simulink model "FaultModel (1)"  (R2018b)
settings: Solver=VariableStepAuto  StartTime=0.0  StopTime=0.05  RelTol=1e-3
undefined symbols (not defined in the file or in its folder): D1, Delta
libraries: powerlib x316
(part 2 of 4)

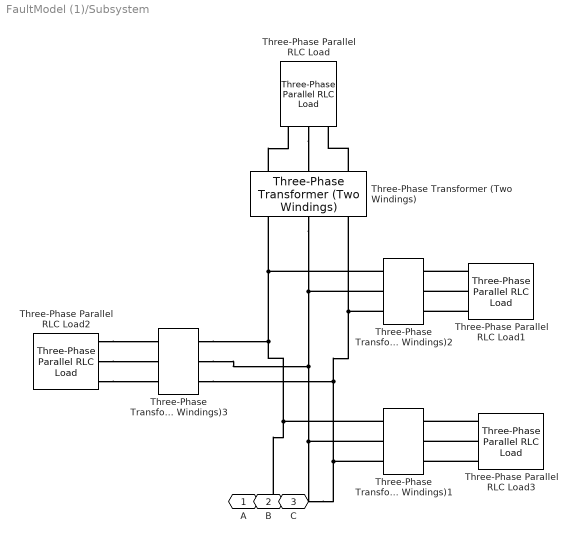
== system FaultModel (1)/Subsystem ==
  Three-Phase Parallel RLC Load{,1..3} (4 alike) : powerlib/Elements/Three-Phase Parallel RLC Load  LConnTagsString=A|B|C  Configuration=Y (grounded)  NominalVoltage=33e3  Vabc=[1e3 1e3 1e3]  Vabcp=[1e3 1e3 1e3]  NominalFrequency=50  UnbalancedPower=off  ActivePower=32.8e6  InductivePower=100  CapacitivePower=100  Pabc=[10e3 9e3 11e3]  QLabc=[100 90 110]  QCabc=[100 90 110]  Pabcp=[10e3 9e3 11e3]  QLabcp=[100 90 110]  QCabcp=[100 90 110]  Measurements=None  LoadType=constant Z
  Three-Phase Transformer (Two Windings){,1..3} (4 alike) : powerlib/Elements/Three-Phase Transformer (Two Windings)  Winding1Connection=Delta (D1)  Winding2Connection=Yg  CoreType=Three single-phase transformers  SetSaturation=off  Hysteresis=off  DataFile='hysteresis'  SetInitialFlux=off  Measurements=None  UNITS=pu  NominalPower=[ 41e6 , 50 ]  Winding1=[ 132e3 , 0.002 , 0.08 ]  Winding2=[ 33e3 , 0.002 , 0.08 ]  Rm=500  Lm=500  L0=0.5  Saturation=[ 0,0 ; 0.0024,1.2 ; 1.0,1.52 ]  InitialFluxes=[ 0.8 , -0.8 , 0.7 ]  BreakLoop=off  DiscreteSolver=Trapezoidal iterative  DataType=off  TransfoNumber=1
  A : PMIOPort  Side=Left
  B : PMIOPort  Port=2  Side=Left
  C : PMIOPort  Port=3  Side=Left
  connections:
  Three-Phase Parallel RLC Load2/LConn3 -- Three-Phase Transformer (Two Windings)3/RConn3
  Three-Phase Parallel RLC Load1/LConn1 -- Three-Phase Transformer (Two Windings)2/RConn1
  Three-Phase Parallel RLC Load1/LConn2 -- Three-Phase Transformer (Two Windings)2/RConn2
  Three-Phase Transformer (Two Windings)1/LConn3 -- C/RConn1 -- Three-Phase Transformer (Two Windings)3/LConn3 -- Three-Phase Transformer (Two Windings)2/LConn3 -- Three-Phase Transformer (Two Windings)/LConn3
  Three-Phase Transformer (Two Windings)/LConn2 -- Three-Phase Transformer (Two Windings)2/LConn2 -- Three-Phase Transformer (Two Windings)3/LConn2 -- B/RConn1 -- Three-Phase Transformer (Two Windings)1/LConn2
  Three-Phase Parallel RLC Load3/LConn2 -- Three-Phase Transformer (Two Windings)1/RConn2
  Three-Phase Transformer (Two Windings)1/LConn1 -- A/RConn1 -- Three-Phase Transformer (Two Windings)3/LConn1 -- Three-Phase Transformer (Two Windings)2/LConn1 -- Three-Phase Transformer (Two Windings)/LConn1
  Three-Phase Parallel RLC Load/LConn2 -- Three-Phase Transformer (Two Windings)/RConn2
  Three-Phase Parallel RLC Load2/LConn2 -- Three-Phase Transformer (Two Windings)3/RConn2
  Three-Phase Transformer (Two Windings)/RConn1 -- Three-Phase Parallel RLC Load/LConn1
  Three-Phase Transformer (Two Windings)/RConn3 -- Three-Phase Parallel RLC Load/LConn3
  Three-Phase Parallel RLC Load2/LConn1 -- Three-Phase Transformer (Two Windings)3/RConn1
  Three-Phase Parallel RLC Load3/LConn3 -- Three-Phase Transformer (Two Windings)1/RConn3
  Three-Phase Parallel RLC Load3/LConn1 -- Three-Phase Transformer (Two Windings)1/RConn1
  Three-Phase Parallel RLC Load1/LConn3 -- Three-Phase Transformer (Two Windings)2/RConn3

== system FaultModel (1)/Subsystem1 ==
  Three-Phase Parallel RLC Load4 : powerlib/Elements/Three-Phase Parallel RLC Load  LConnTagsString=A|B|C  Configuration=Y (grounded)  NominalVoltage=33e3  Vabc=[1e3 1e3 1e3]  Vabcp=[1e3 1e3 1e3]  NominalFrequency=50  UnbalancedPower=off  ActivePower=60e6  InductivePower=100  CapacitivePower=100  Pabc=[10e3 9e3 11e3]  QLabc=[100 90 110]  QCabc=[100 90 110]  Pabcp=[10e3 9e3 11e3]  QLabcp=[100 90 110]  QCabcp=[100 90 110]  Measurements=None  LoadType=constant Z
  Three-Phase Parallel RLC Load5 : powerlib/Elements/Three-Phase Parallel RLC Load  LConnTagsString=A|B|C  Configuration=Y (grounded)  NominalVoltage=33e3  Vabc=[1e3 1e3 1e3]  Vabcp=[1e3 1e3 1e3]  NominalFrequency=50  UnbalancedPower=off  ActivePower=60e6  InductivePower=100  CapacitivePower=100  Pabc=[10e3 9e3 11e3]  QLabc=[100 90 110]  QCabc=[100 90 110]  Pabcp=[10e3 9e3 11e3]  QLabcp=[100 90 110]  QCabcp=[100 90 110]  Measurements=None  LoadType=constant Z
  Three-Phase Transformer (Two Windings)4 : powerlib/Elements/Three-Phase Transformer (Two Windings)  Winding1Connection=Delta (D1)  Winding2Connection=Yg  CoreType=Three single-phase transformers  SetSaturation=off  Hysteresis=off  DataFile='hysteresis'  SetInitialFlux=off  Measurements=None  UNITS=pu  NominalPower=[ 75e6 , 50 ]  Winding1=[ 132e3 , 0.002 , 0.08 ]  Winding2=[ 33e3 , 0.002 , 0.08 ]  Rm=500  Lm=500  L0=0.5  Saturation=[ 0,0 ; 0.0024,1.2 ; 1.0,1.52 ]  InitialFluxes=[ 0.8 , -0.8 , 0.7 ]  BreakLoop=off  DiscreteSolver=Trapezoidal iterative  DataType=off  TransfoNumber=1
  Three-Phase Transformer (Two Windings)5 : powerlib/Elements/Three-Phase Transformer (Two Windings)  Winding1Connection=Delta (D1)  Winding2Connection=Yg  CoreType=Three single-phase transformers  SetSaturation=off  Hysteresis=off  DataFile='hysteresis'  SetInitialFlux=off  Measurements=None  UNITS=pu  NominalPower=[ 75e6 , 50 ]  Winding1=[ 132e3 , 0.002 , 0.08 ]  Winding2=[ 33e3 , 0.002 , 0.08 ]  Rm=500  Lm=500  L0=0.5  Saturation=[ 0,0 ; 0.0024,1.2 ; 1.0,1.52 ]  InitialFluxes=[ 0.8 , -0.8 , 0.7 ]  BreakLoop=off  DiscreteSolver=Trapezoidal iterative  DataType=off  TransfoNumber=1
  A : PMIOPort  Side=Left
  B : PMIOPort  Port=2  Side=Left
  C : PMIOPort  Port=3  Side=Left
  connections:
  Three-Phase Parallel RLC Load4/LConn2 -- Three-Phase Transformer (Two Windings)5/RConn2
  Three-Phase Parallel RLC Load5/LConn1 -- Three-Phase Transformer (Two Windings)4/RConn1
  Three-Phase Transformer (Two Windings)5/LConn3 -- C/RConn1 -- Three-Phase Transformer (Two Windings)4/LConn3
  Three-Phase Transformer (Two Windings)4/LConn2 -- B/RConn1 -- Three-Phase Transformer (Two Windings)5/LConn2
  Three-Phase Parallel RLC Load4/LConn1 -- Three-Phase Transformer (Two Windings)5/RConn1
  Three-Phase Transformer (Two Windings)4/LConn1 -- A/RConn1 -- Three-Phase Transformer (Two Windings)5/LConn1
  Three-Phase Parallel RLC Load5/LConn2 -- Three-Phase Transformer (Two Windings)4/RConn2
  Three-Phase Parallel RLC Load5/LConn3 -- Three-Phase Transformer (Two Windings)4/RConn3
  Three-Phase Parallel RLC Load4/LConn3 -- Three-Phase Transformer (Two Windings)5/RConn3

== system FaultModel (1)/Subsystem10 ==
  Three-Phase Parallel RLC Load34 : powerlib/Elements/Three-Phase Parallel RLC Load  LConnTagsString=A|B|C  Configuration=Y (grounded)  NominalVoltage=33e3  Vabc=[1e3 1e3 1e3]  Vabcp=[1e3 1e3 1e3]  NominalFrequency=50  UnbalancedPower=off  ActivePower=96e6  InductivePower=100  CapacitivePower=100  Pabc=[10e3 9e3 11e3]  QLabc=[100 90 110]  QCabc=[100 90 110]  Pabcp=[10e3 9e3 11e3]  QLabcp=[100 90 110]  QCabcp=[100 90 110]  Measurements=None  LoadType=constant Z
  Three-Phase Parallel RLC Load35 : powerlib/Elements/Three-Phase Parallel RLC Load  LConnTagsString=A|B|C  Configuration=Y (grounded)  NominalVoltage=33e3  Vabc=[1e3 1e3 1e3]  Vabcp=[1e3 1e3 1e3]  NominalFrequency=50  UnbalancedPower=off  ActivePower=96e6  InductivePower=100  CapacitivePower=100  Pabc=[10e3 9e3 11e3]  QLabc=[100 90 110]  QCabc=[100 90 110]  Pabcp=[10e3 9e3 11e3]  QLabcp=[100 90 110]  QCabcp=[100 90 110]  Measurements=None  LoadType=constant Z
  Three-Phase Transformer (Two Windings)34 : powerlib/Elements/Three-Phase Transformer (Two Windings)  Winding1Connection=Delta (D1)  Winding2Connection=Yg  CoreType=Three single-phase transformers  SetSaturation=off  Hysteresis=off  DataFile='hysteresis'  SetInitialFlux=off  Measurements=None  UNITS=pu  NominalPower=[120e6 , 50 ]  Winding1=[ 132e3 , 0.002 , 0.08 ]  Winding2=[ 33e3 , 0.002 , 0.08 ]  Rm=500  Lm=500  L0=0.5  Saturation=[ 0,0 ; 0.0024,1.2 ; 1.0,1.52 ]  InitialFluxes=[ 0.8 , -0.8 , 0.7 ]  BreakLoop=off  DiscreteSolver=Trapezoidal iterative  DataType=off  TransfoNumber=1
  Three-Phase Transformer (Two Windings)35 : powerlib/Elements/Three-Phase Transformer (Two Windings)  Winding1Connection=Delta (D1)  Winding2Connection=Yg  CoreType=Three single-phase transformers  SetSaturation=off  Hysteresis=off  DataFile='hysteresis'  SetInitialFlux=off  Measurements=None  UNITS=pu  NominalPower=[120e6 , 50 ]  Winding1=[ 132e3 , 0.002 , 0.08 ]  Winding2=[ 33e3 , 0.002 , 0.08 ]  Rm=500  Lm=500  L0=0.5  Saturation=[ 0,0 ; 0.0024,1.2 ; 1.0,1.52 ]  InitialFluxes=[ 0.8 , -0.8 , 0.7 ]  BreakLoop=off  DiscreteSolver=Trapezoidal iterative  DataType=off  TransfoNumber=1
  A : PMIOPort  Side=Left
  B : PMIOPort  Port=2  Side=Left
  C : PMIOPort  Port=3  Side=Left
  connections:
  Three-Phase Parallel RLC Load35/LConn3 -- Three-Phase Transformer (Two Windings)35/RConn3
  Three-Phase Transformer (Two Windings)34/LConn3 -- C/RConn1 -- Three-Phase Transformer (Two Windings)35/LConn3
  Three-Phase Parallel RLC Load34/LConn2 -- Three-Phase Transformer (Two Windings)34/RConn2
  Three-Phase Transformer (Two Windings)34/LConn2 -- B/RConn1 -- Three-Phase Transformer (Two Windings)35/LConn2
  Three-Phase Parallel RLC Load34/LConn3 -- Three-Phase Transformer (Two Windings)34/RConn3
  Three-Phase Parallel RLC Load35/LConn2 -- Three-Phase Transformer (Two Windings)35/RConn2
  Three-Phase Parallel RLC Load35/LConn1 -- Three-Phase Transformer (Two Windings)35/RConn1
  Three-Phase Parallel RLC Load34/LConn1 -- Three-Phase Transformer (Two Windings)34/RConn1
  Three-Phase Transformer (Two Windings)34/LConn1 -- A/RConn1 -- Three-Phase Transformer (Two Windings)35/LConn1

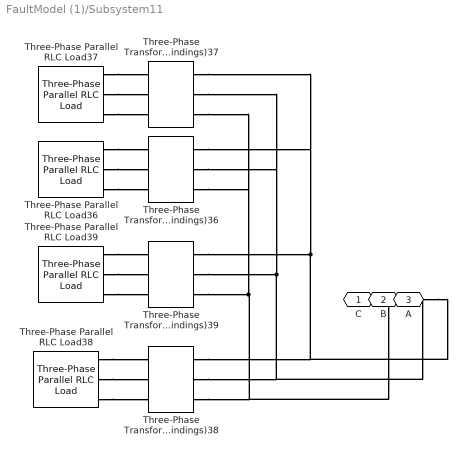
== system FaultModel (1)/Subsystem11 ==
  Three-Phase Parallel RLC Load{36..39} (4 alike) : powerlib/Elements/Three-Phase Parallel RLC Load  LConnTagsString=A|B|C  Configuration=Y (grounded)  NominalVoltage=33e3  Vabc=[1e3 1e3 1e3]  Vabcp=[1e3 1e3 1e3]  NominalFrequency=50  UnbalancedPower=off  ActivePower=32.8e6  InductivePower=100  CapacitivePower=100  Pabc=[10e3 9e3 11e3]  QLabc=[100 90 110]  QCabc=[100 90 110]  Pabcp=[10e3 9e3 11e3]  QLabcp=[100 90 110]  QCabcp=[100 90 110]  Measurements=None  LoadType=constant Z
  Three-Phase Transformer (Two Windings){36..39} (4 alike) : powerlib/Elements/Three-Phase Transformer (Two Windings)  Winding1Connection=Delta (D1)  Winding2Connection=Yg  CoreType=Three single-phase transformers  SetSaturation=off  Hysteresis=off  DataFile='hysteresis'  SetInitialFlux=off  Measurements=None  UNITS=pu  NominalPower=[41e6 , 50 ]  Winding1=[ 132e3 , 0.002 , 0.08 ]  Winding2=[ 33e3 , 0.002 , 0.08 ]  Rm=500  Lm=500  L0=0.5  Saturation=[ 0,0 ; 0.0024,1.2 ; 1.0,1.52 ]  InitialFluxes=[ 0.8 , -0.8 , 0.7 ]  BreakLoop=off  DiscreteSolver=Trapezoidal iterative  DataType=off  TransfoNumber=1
  C : PMIOPort  Side=Left
  B : PMIOPort  Port=2  Side=Left
  A : PMIOPort  Port=3  Side=Left
  connections:
  Three-Phase Transformer (Two Windings)39/LConn1 -- Three-Phase Transformer (Two Windings)37/LConn1 -- Three-Phase Transformer (Two Windings)36/LConn1 -- A/RConn1 -- Three-Phase Transformer (Two Windings)38/LConn1
  Three-Phase Parallel RLC Load38/LConn3 -- Three-Phase Transformer (Two Windings)38/RConn3
  Three-Phase Parallel RLC Load36/LConn3 -- Three-Phase Transformer (Two Windings)36/RConn3
  Three-Phase Parallel RLC Load36/LConn1 -- Three-Phase Transformer (Two Windings)36/RConn1
  Three-Phase Parallel RLC Load37/LConn1 -- Three-Phase Transformer (Two Windings)37/RConn1
  Three-Phase Transformer (Two Windings)39/LConn3 -- Three-Phase Transformer (Two Windings)37/LConn3 -- Three-Phase Transformer (Two Windings)36/LConn3 -- C/RConn1 -- Three-Phase Transformer (Two Windings)38/LConn3
  Three-Phase Parallel RLC Load37/LConn3 -- Three-Phase Transformer (Two Windings)37/RConn3
  Three-Phase Transformer (Two Windings)39/LConn2 -- Three-Phase Transformer (Two Windings)37/LConn2 -- Three-Phase Transformer (Two Windings)36/LConn2 -- B/RConn1 -- Three-Phase Transformer (Two Windings)38/LConn2
  Three-Phase Parallel RLC Load39/LConn1 -- Three-Phase Transformer (Two Windings)39/RConn1
  Three-Phase Parallel RLC Load38/LConn2 -- Three-Phase Transformer (Two Windings)38/RConn2
  Three-Phase Parallel RLC Load38/LConn1 -- Three-Phase Transformer (Two Windings)38/RConn1
  Three-Phase Parallel RLC Load39/LConn2 -- Three-Phase Transformer (Two Windings)39/RConn2
  Three-Phase Parallel RLC Load36/LConn2 -- Three-Phase Transformer (Two Windings)36/RConn2
  Three-Phase Parallel RLC Load37/LConn2 -- Three-Phase Transformer (Two Windings)37/RConn2
  Three-Phase Parallel RLC Load39/LConn3 -- Three-Phase Transformer (Two Windings)39/RConn3

== system FaultModel (1)/Subsystem12 ==
  Three-Phase Parallel RLC Load40 : powerlib/Elements/Three-Phase Parallel RLC Load  LConnTagsString=A|B|C  Configuration=Y (grounded)  NominalVoltage=33e3  Vabc=[1e3 1e3 1e3]  Vabcp=[1e3 1e3 1e3]  NominalFrequency=50  UnbalancedPower=off  ActivePower=32.8e6  InductivePower=100  CapacitivePower=100  Pabc=[10e3 9e3 11e3]  QLabc=[100 90 110]  QCabc=[100 90 110]  Pabcp=[10e3 9e3 11e3]  QLabcp=[100 90 110]  QCabcp=[100 90 110]  Measurements=None  LoadType=constant Z
  Three-Phase Parallel RLC Load41 : powerlib/Elements/Three-Phase Parallel RLC Load  LConnTagsString=A|B|C  Configuration=Y (grounded)  NominalVoltage=33e3  Vabc=[1e3 1e3 1e3]  Vabcp=[1e3 1e3 1e3]  NominalFrequency=50  UnbalancedPower=off  ActivePower=40e6  InductivePower=100  CapacitivePower=100  Pabc=[10e3 9e3 11e3]  QLabc=[100 90 110]  QCabc=[100 90 110]  Pabcp=[10e3 9e3 11e3]  QLabcp=[100 90 110]  QCabcp=[100 90 110]  Measurements=None  LoadType=constant Z
  Three-Phase Parallel RLC Load42 : powerlib/Elements/Three-Phase Parallel RLC Load  LConnTagsString=A|B|C  Configuration=Y (grounded)  NominalVoltage=33e3  Vabc=[1e3 1e3 1e3]  Vabcp=[1e3 1e3 1e3]  NominalFrequency=50  UnbalancedPower=off  ActivePower=40e6  InductivePower=100  CapacitivePower=100  Pabc=[10e3 9e3 11e3]  QLabc=[100 90 110]  QCabc=[100 90 110]  Pabcp=[10e3 9e3 11e3]  QLabcp=[100 90 110]  QCabcp=[100 90 110]  Measurements=None  LoadType=constant Z
  Three-Phase Transformer (Two Windings)40 : powerlib/Elements/Three-Phase Transformer (Two Windings)  Winding1Connection=Delta (D1)  Winding2Connection=Yg  CoreType=Three single-phase transformers  SetSaturation=off  Hysteresis=off  DataFile='hysteresis'  SetInitialFlux=off  Measurements=None  UNITS=pu  NominalPower=[41e6 , 50 ]  Winding1=[ 132e3 , 0.002 , 0.08 ]  Winding2=[ 33e3 , 0.002 , 0.08 ]  Rm=500  Lm=500  L0=0.5  Saturation=[ 0,0 ; 0.0024,1.2 ; 1.0,1.52 ]  InitialFluxes=[ 0.8 , -0.8 , 0.7 ]  BreakLoop=off  DiscreteSolver=Trapezoidal iterative  DataType=off  TransfoNumber=1
  Three-Phase Transformer (Two Windings)41 : powerlib/Elements/Three-Phase Transformer (Two Windings)  Winding1Connection=Delta (D1)  Winding2Connection=Yg  CoreType=Three single-phase transformers  SetSaturation=off  Hysteresis=off  DataFile='hysteresis'  SetInitialFlux=off  Measurements=None  UNITS=pu  NominalPower=[50e6 , 50 ]  Winding1=[ 132e3 , 0.002 , 0.08 ]  Winding2=[ 33e3 , 0.002 , 0.08 ]  Rm=500  Lm=500  L0=0.5  Saturation=[ 0,0 ; 0.0024,1.2 ; 1.0,1.52 ]  InitialFluxes=[ 0.8 , -0.8 , 0.7 ]  BreakLoop=off  DiscreteSolver=Trapezoidal iterative  DataType=off  TransfoNumber=1
  Three-Phase Transformer (Two Windings)42 : powerlib/Elements/Three-Phase Transformer (Two Windings)  Winding1Connection=Delta (D1)  Winding2Connection=Yg  CoreType=Three single-phase transformers  SetSaturation=off  Hysteresis=off  DataFile='hysteresis'  SetInitialFlux=off  Measurements=None  UNITS=pu  NominalPower=[50e6 , 50 ]  Winding1=[ 132e3 , 0.002 , 0.08 ]  Winding2=[ 33e3 , 0.002 , 0.08 ]  Rm=500  Lm=500  L0=0.5  Saturation=[ 0,0 ; 0.0024,1.2 ; 1.0,1.52 ]  InitialFluxes=[ 0.8 , -0.8 , 0.7 ]  BreakLoop=off  DiscreteSolver=Trapezoidal iterative  DataType=off  TransfoNumber=1
  A : PMIOPort  Side=Left
  B : PMIOPort  Port=2  Side=Left
  C : PMIOPort  Port=3  Side=Left
  connections:
  Three-Phase Parallel RLC Load40/LConn2 -- Three-Phase Transformer (Two Windings)40/RConn2
  Three-Phase Parallel RLC Load42/LConn2 -- Three-Phase Transformer (Two Windings)42/RConn2
  Three-Phase Transformer (Two Windings)42/LConn2 -- Three-Phase Transformer (Two Windings)41/LConn2 -- Three-Phase Transformer (Two Windings)40/LConn2 -- B/RConn1
  Three-Phase Transformer (Two Windings)41/LConn3 -- Three-Phase Transformer (Two Windings)42/LConn3 -- C/RConn1 -- Three-Phase Transformer (Two Windings)40/LConn3
  Three-Phase Parallel RLC Load40/LConn1 -- Three-Phase Transformer (Two Windings)40/RConn1
  Three-Phase Parallel RLC Load41/LConn2 -- Three-Phase Transformer (Two Windings)41/RConn2
  Three-Phase Parallel RLC Load40/LConn3 -- Three-Phase Transformer (Two Windings)40/RConn3
  Three-Phase Parallel RLC Load42/LConn1 -- Three-Phase Transformer (Two Windings)42/RConn1
  Three-Phase Parallel RLC Load41/LConn3 -- Three-Phase Transformer (Two Windings)41/RConn3
  Three-Phase Parallel RLC Load42/LConn3 -- Three-Phase Transformer (Two Windings)42/RConn3
  Three-Phase Transformer (Two Windings)42/LConn1 -- A/RConn1 -- Three-Phase Transformer (Two Windings)41/LConn1 -- Three-Phase Transformer (Two Windings)40/LConn1
  Three-Phase Parallel RLC Load41/LConn1 -- Three-Phase Transformer (Two Windings)41/RConn1

== system FaultModel (1)/Subsystem13 ==
  Three-Phase Parallel RLC Load43 : powerlib/Elements/Three-Phase Parallel RLC Load  LConnTagsString=A|B|C  Configuration=Y (grounded)  NominalVoltage=33e3  Vabc=[1e3 1e3 1e3]  Vabcp=[1e3 1e3 1e3]  NominalFrequency=50  UnbalancedPower=off  ActivePower=60e6  InductivePower=100  CapacitivePower=100  Pabc=[10e3 9e3 11e3]  QLabc=[100 90 110]  QCabc=[100 90 110]  Pabcp=[10e3 9e3 11e3]  QLabcp=[100 90 110]  QCabcp=[100 90 110]  Measurements=None  LoadType=constant Z
  Three-Phase Parallel RLC Load44 : powerlib/Elements/Three-Phase Parallel RLC Load  LConnTagsString=A|B|C  Configuration=Y (grounded)  NominalVoltage=33e3  Vabc=[1e3 1e3 1e3]  Vabcp=[1e3 1e3 1e3]  NominalFrequency=50  UnbalancedPower=off  ActivePower=60e6  InductivePower=100  CapacitivePower=100  Pabc=[10e3 9e3 11e3]  QLabc=[100 90 110]  QCabc=[100 90 110]  Pabcp=[10e3 9e3 11e3]  QLabcp=[100 90 110]  QCabcp=[100 90 110]  Measurements=None  LoadType=constant Z
  Three-Phase Parallel RLC Load45 : powerlib/Elements/Three-Phase Parallel RLC Load  LConnTagsString=A|B|C  Configuration=Y (grounded)  NominalVoltage=33e3  Vabc=[1e3 1e3 1e3]  Vabcp=[1e3 1e3 1e3]  NominalFrequency=50  UnbalancedPower=off  ActivePower=60e6  InductivePower=100  CapacitivePower=100  Pabc=[10e3 9e3 11e3]  QLabc=[100 90 110]  QCabc=[100 90 110]  Pabcp=[10e3 9e3 11e3]  QLabcp=[100 90 110]  QCabcp=[100 90 110]  Measurements=None  LoadType=constant Z
  Three-Phase Transformer (Two Windings)43 : powerlib/Elements/Three-Phase Transformer (Two Windings)  Winding1Connection=Delta (D1)  Winding2Connection=Yg  CoreType=Three single-phase transformers  SetSaturation=off  Hysteresis=off  DataFile='hysteresis'  SetInitialFlux=off  Measurements=None  UNITS=pu  NominalPower=[75e6 , 50 ]  Winding1=[ 132e3 , 0.002 , 0.08 ]  Winding2=[ 33e3 , 0.002 , 0.08 ]  Rm=500  Lm=500  L0=0.5  Saturation=[ 0,0 ; 0.0024,1.2 ; 1.0,1.52 ]  InitialFluxes=[ 0.8 , -0.8 , 0.7 ]  BreakLoop=off  DiscreteSolver=Trapezoidal iterative  DataType=off  TransfoNumber=1
  Three-Phase Transformer (Two Windings)44 : powerlib/Elements/Three-Phase Transformer (Two Windings)  Winding1Connection=Delta (D1)  Winding2Connection=Yg  CoreType=Three single-phase transformers  SetSaturation=off  Hysteresis=off  DataFile='hysteresis'  SetInitialFlux=off  Measurements=None  UNITS=pu  NominalPower=[75e6 , 50 ]  Winding1=[ 132e3 , 0.002 , 0.08 ]  Winding2=[ 33e3 , 0.002 , 0.08 ]  Rm=500  Lm=500  L0=0.5  Saturation=[ 0,0 ; 0.0024,1.2 ; 1.0,1.52 ]  InitialFluxes=[ 0.8 , -0.8 , 0.7 ]  BreakLoop=off  DiscreteSolver=Trapezoidal iterative  DataType=off  TransfoNumber=1
  Three-Phase Transformer (Two Windings)45 : powerlib/Elements/Three-Phase Transformer (Two Windings)  Winding1Connection=Delta (D1)  Winding2Connection=Yg  CoreType=Three single-phase transformers  SetSaturation=off  Hysteresis=off  DataFile='hysteresis'  SetInitialFlux=off  Measurements=None  UNITS=pu  NominalPower=[75e6 , 50 ]  Winding1=[ 132e3 , 0.002 , 0.08 ]  Winding2=[ 33e3 , 0.002 , 0.08 ]  Rm=500  Lm=500  L0=0.5  Saturation=[ 0,0 ; 0.0024,1.2 ; 1.0,1.52 ]  InitialFluxes=[ 0.8 , -0.8 , 0.7 ]  BreakLoop=off  DiscreteSolver=Trapezoidal iterative  DataType=off  TransfoNumber=1
  A : PMIOPort  Side=Left
  B : PMIOPort  Port=2  Side=Left
  C : PMIOPort  Port=3  Side=Left
  connections:
  Three-Phase Parallel RLC Load43/LConn3 -- Three-Phase Transformer (Two Windings)43/RConn3
  Three-Phase Transformer (Two Windings)43/LConn2 -- B/RConn1 -- Three-Phase Transformer (Two Windings)44/LConn2 -- Three-Phase Transformer (Two Windings)45/LConn2
  Three-Phase Parallel RLC Load43/LConn2 -- Three-Phase Transformer (Two Windings)43/RConn2
  Three-Phase Transformer (Two Windings)43/LConn1 -- A/RConn1 -- Three-Phase Transformer (Two Windings)44/LConn1 -- Three-Phase Transformer (Two Windings)45/LConn1
  Three-Phase Transformer (Two Windings)43/LConn3 -- C/RConn1 -- Three-Phase Transformer (Two Windings)44/LConn3 -- Three-Phase Transformer (Two Windings)45/LConn3
  Three-Phase Parallel RLC Load44/LConn1 -- Three-Phase Transformer (Two Windings)44/RConn1
  Three-Phase Parallel RLC Load43/LConn1 -- Three-Phase Transformer (Two Windings)43/RConn1
  Three-Phase Parallel RLC Load45/LConn1 -- Three-Phase Transformer (Two Windings)45/RConn1
  Three-Phase Parallel RLC Load44/LConn2 -- Three-Phase Transformer (Two Windings)44/RConn2
  Three-Phase Parallel RLC Load45/LConn3 -- Three-Phase Transformer (Two Windings)45/RConn3
  Three-Phase Parallel RLC Load44/LConn3 -- Three-Phase Transformer (Two Windings)44/RConn3
  Three-Phase Parallel RLC Load45/LConn2 -- Three-Phase Transformer (Two Windings)45/RConn2

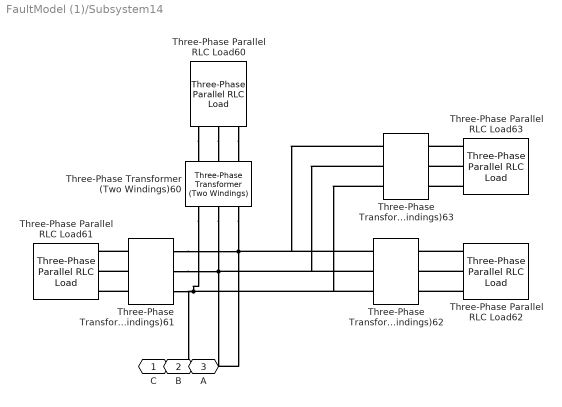
== system FaultModel (1)/Subsystem14 ==
  Three-Phase Parallel RLC Load60 : powerlib/Elements/Three-Phase Parallel RLC Load  LConnTagsString=A|B|C  Configuration=Y (grounded)  NominalVoltage=33e3  Vabc=[1e3 1e3 1e3]  Vabcp=[1e3 1e3 1e3]  NominalFrequency=50  UnbalancedPower=off  ActivePower=60e6  InductivePower=100  CapacitivePower=100  Pabc=[10e3 9e3 11e3]  QLabc=[100 90 110]  QCabc=[100 90 110]  Pabcp=[10e3 9e3 11e3]  QLabcp=[100 90 110]  QCabcp=[100 90 110]  Measurements=None  LoadType=constant Z
  Three-Phase Parallel RLC Load61 : powerlib/Elements/Three-Phase Parallel RLC Load  LConnTagsString=A|B|C  Configuration=Y (grounded)  NominalVoltage=33e3  Vabc=[1e3 1e3 1e3]  Vabcp=[1e3 1e3 1e3]  NominalFrequency=50  UnbalancedPower=off  ActivePower=60e6  InductivePower=100  CapacitivePower=100  Pabc=[10e3 9e3 11e3]  QLabc=[100 90 110]  QCabc=[100 90 110]  Pabcp=[10e3 9e3 11e3]  QLabcp=[100 90 110]  QCabcp=[100 90 110]  Measurements=None  LoadType=constant Z
  Three-Phase Parallel RLC Load62 : powerlib/Elements/Three-Phase Parallel RLC Load  LConnTagsString=A|B|C  Configuration=Y (grounded)  NominalVoltage=33e3  Vabc=[1e3 1e3 1e3]  Vabcp=[1e3 1e3 1e3]  NominalFrequency=50  UnbalancedPower=off  ActivePower=32.8e6  InductivePower=100  CapacitivePower=100  Pabc=[10e3 9e3 11e3]  QLabc=[100 90 110]  QCabc=[100 90 110]  Pabcp=[10e3 9e3 11e3]  QLabcp=[100 90 110]  QCabcp=[100 90 110]  Measurements=None  LoadType=constant Z
  Three-Phase Parallel RLC Load63 : powerlib/Elements/Three-Phase Parallel RLC Load  LConnTagsString=A|B|C  Configuration=Y (grounded)  NominalVoltage=33e3  Vabc=[1e3 1e3 1e3]  Vabcp=[1e3 1e3 1e3]  NominalFrequency=50  UnbalancedPower=off  ActivePower=16e6  InductivePower=100  CapacitivePower=100  Pabc=[10e3 9e3 11e3]  QLabc=[100 90 110]  QCabc=[100 90 110]  Pabcp=[10e3 9e3 11e3]  QLabcp=[100 90 110]  QCabcp=[100 90 110]  Measurements=None  LoadType=constant Z
  Three-Phase Transformer (Two Windings)60 : powerlib/Elements/Three-Phase Transformer (Two Windings)  Winding1Connection=Delta (D1)  Winding2Connection=Yg  CoreType=Three single-phase transformers  SetSaturation=off  Hysteresis=off  DataFile='hysteresis'  SetInitialFlux=off  Measurements=None  UNITS=pu  NominalPower=[75e6 , 50 ]  Winding1=[ 132e3 , 0.002 , 0.08 ]  Winding2=[ 33e3 , 0.002 , 0.08 ]  Rm=500  Lm=500  L0=0.5  Saturation=[ 0,0 ; 0.0024,1.2 ; 1.0,1.52 ]  InitialFluxes=[ 0.8 , -0.8 , 0.7 ]  BreakLoop=off  DiscreteSolver=Trapezoidal iterative  DataType=off  TransfoNumber=1
  Three-Phase Transformer (Two Windings)61 : powerlib/Elements/Three-Phase Transformer (Two Windings)  Winding1Connection=Delta (D1)  Winding2Connection=Yg  CoreType=Three single-phase transformers  SetSaturation=off  Hysteresis=off  DataFile='hysteresis'  SetInitialFlux=off  Measurements=None  UNITS=pu  NominalPower=[75e6 , 50 ]  Winding1=[ 132e3 , 0.002 , 0.08 ]  Winding2=[ 33e3 , 0.002 , 0.08 ]  Rm=500  Lm=500  L0=0.5  Saturation=[ 0,0 ; 0.0024,1.2 ; 1.0,1.52 ]  InitialFluxes=[ 0.8 , -0.8 , 0.7 ]  BreakLoop=off  DiscreteSolver=Trapezoidal iterative  DataType=off  TransfoNumber=1
  Three-Phase Transformer (Two Windings)62 : powerlib/Elements/Three-Phase Transformer (Two Windings)  Winding1Connection=Delta (D1)  Winding2Connection=Yg  CoreType=Three single-phase transformers  SetSaturation=off  Hysteresis=off  DataFile='hysteresis'  SetInitialFlux=off  Measurements=None  UNITS=pu  NominalPower=[41e6 , 50 ]  Winding1=[ 132e3 , 0.002 , 0.08 ]  Winding2=[ 33e3 , 0.002 , 0.08 ]  Rm=500  Lm=500  L0=0.5  Saturation=[ 0,0 ; 0.0024,1.2 ; 1.0,1.52 ]  InitialFluxes=[ 0.8 , -0.8 , 0.7 ]  BreakLoop=off  DiscreteSolver=Trapezoidal iterative  DataType=off  TransfoNumber=1
  Three-Phase Transformer (Two Windings)63 : powerlib/Elements/Three-Phase Transformer (Two Windings)  Winding1Connection=Delta (D1)  Winding2Connection=Yg  CoreType=Three single-phase transformers  SetSaturation=off  Hysteresis=off  DataFile='hysteresis'  SetInitialFlux=off  Measurements=None  UNITS=pu  NominalPower=[20e6 , 50 ]  Winding1=[ 132e3 , 0.002 , 0.08 ]  Winding2=[ 33e3 , 0.002 , 0.08 ]  Rm=500  Lm=500  L0=0.5  Saturation=[ 0,0 ; 0.0024,1.2 ; 1.0,1.52 ]  InitialFluxes=[ 0.8 , -0.8 , 0.7 ]  BreakLoop=off  DiscreteSolver=Trapezoidal iterative  DataType=off  TransfoNumber=1
  C : PMIOPort  Side=Left
  B : PMIOPort  Port=2  Side=Left
  A : PMIOPort  Port=3  Side=Left
  connections:
  Three-Phase Parallel RLC Load62/LConn2 -- Three-Phase Transformer (Two Windings)62/RConn2
  Three-Phase Parallel RLC Load60/LConn3 -- Three-Phase Transformer (Two Windings)60/RConn1
  Three-Phase Parallel RLC Load62/LConn3 -- Three-Phase Transformer (Two Windings)62/RConn3
  Three-Phase Transformer (Two Windings)60/LConn2 -- B/RConn1 -- Three-Phase Transformer (Two Windings)63/LConn2 -- Three-Phase Transformer (Two Windings)62/LConn2 -- Three-Phase Transformer (Two Windings)61/LConn2
  Three-Phase Parallel RLC Load60/LConn2 -- Three-Phase Transformer (Two Windings)60/RConn2
  Three-Phase Transformer (Two Windings)61/RConn2 -- Three-Phase Parallel RLC Load61/LConn2
  Three-Phase Parallel RLC Load60/LConn1 -- Three-Phase Transformer (Two Windings)60/RConn3
  Three-Phase Transformer (Two Windings)60/LConn3 -- Three-Phase Transformer (Two Windings)61/LConn3 -- C/RConn1 -- Three-Phase Transformer (Two Windings)63/LConn3 -- Three-Phase Transformer (Two Windings)62/LConn3
  Three-Phase Parallel RLC Load62/LConn1 -- Three-Phase Transformer (Two Windings)62/RConn1
  Three-Phase Transformer (Two Windings)60/LConn1 -- A/RConn1 -- Three-Phase Transformer (Two Windings)63/LConn1 -- Three-Phase Transformer (Two Windings)62/LConn1 -- Three-Phase Transformer (Two Windings)61/LConn1
  Three-Phase Parallel RLC Load63/LConn1 -- Three-Phase Transformer (Two Windings)63/RConn1
  Three-Phase Transformer (Two Windings)61/RConn3 -- Three-Phase Parallel RLC Load61/LConn3
  Three-Phase Parallel RLC Load63/LConn3 -- Three-Phase Transformer (Two Windings)63/RConn3
  Three-Phase Transformer (Two Windings)61/RConn1 -- Three-Phase Parallel RLC Load61/LConn1
  Three-Phase Parallel RLC Load63/LConn2 -- Three-Phase Transformer (Two Windings)63/RConn2

== system FaultModel (1)/Subsystem15 ==
  Three-Phase Parallel RLC Load58 : powerlib/Elements/Three-Phase Parallel RLC Load  LConnTagsString=A|B|C  Configuration=Y (grounded)  NominalVoltage=33e3  Vabc=[1e3 1e3 1e3]  Vabcp=[1e3 1e3 1e3]  NominalFrequency=50  UnbalancedPower=off  ActivePower=96e6  InductivePower=100  CapacitivePower=100  Pabc=[10e3 9e3 11e3]  QLabc=[100 90 110]  QCabc=[100 90 110]  Pabcp=[10e3 9e3 11e3]  QLabcp=[100 90 110]  QCabcp=[100 90 110]  Measurements=None  LoadType=constant Z
  Three-Phase Parallel RLC Load59 : powerlib/Elements/Three-Phase Parallel RLC Load  LConnTagsString=A|B|C  Configuration=Y (grounded)  NominalVoltage=33e3  Vabc=[1e3 1e3 1e3]  Vabcp=[1e3 1e3 1e3]  NominalFrequency=50  UnbalancedPower=off  ActivePower=96e6  InductivePower=100  CapacitivePower=100  Pabc=[10e3 9e3 11e3]  QLabc=[100 90 110]  QCabc=[100 90 110]  Pabcp=[10e3 9e3 11e3]  QLabcp=[100 90 110]  QCabcp=[100 90 110]  Measurements=None  LoadType=constant Z
  Three-Phase Transformer (Two Windings)58 : powerlib/Elements/Three-Phase Transformer (Two Windings)  Winding1Connection=Delta (D1)  Winding2Connection=Yg  CoreType=Three single-phase transformers  SetSaturation=off  Hysteresis=off  DataFile='hysteresis'  SetInitialFlux=off  Measurements=None  UNITS=pu  NominalPower=[120e6 , 50 ]  Winding1=[ 132e3 , 0.002 , 0.08 ]  Winding2=[ 33e3 , 0.002 , 0.08 ]  Rm=500  Lm=500  L0=0.5  Saturation=[ 0,0 ; 0.0024,1.2 ; 1.0,1.52 ]  InitialFluxes=[ 0.8 , -0.8 , 0.7 ]  BreakLoop=off  DiscreteSolver=Trapezoidal iterative  DataType=off  TransfoNumber=1
  Three-Phase Transformer (Two Windings)59 : powerlib/Elements/Three-Phase Transformer (Two Windings)  Winding1Connection=Delta (D1)  Winding2Connection=Yg  CoreType=Three single-phase transformers  SetSaturation=off  Hysteresis=off  DataFile='hysteresis'  SetInitialFlux=off  Measurements=None  UNITS=pu  NominalPower=[120e6 , 50 ]  Winding1=[ 132e3 , 0.002 , 0.08 ]  Winding2=[ 33e3 , 0.002 , 0.08 ]  Rm=500  Lm=500  L0=0.5  Saturation=[ 0,0 ; 0.0024,1.2 ; 1.0,1.52 ]  InitialFluxes=[ 0.8 , -0.8 , 0.7 ]  BreakLoop=off  DiscreteSolver=Trapezoidal iterative  DataType=off  TransfoNumber=1
  C : PMIOPort  Side=Left
  B : PMIOPort  Port=2  Side=Left
  A : PMIOPort  Port=3  Side=Left
  connections:
  Three-Phase Transformer (Two Windings)58/LConn3 -- C/RConn1 -- Three-Phase Transformer (Two Windings)59/LConn3
  Three-Phase Parallel RLC Load58/LConn1 -- Three-Phase Transformer (Two Windings)58/RConn3
  Three-Phase Parallel RLC Load59/LConn3 -- Three-Phase Transformer (Two Windings)59/RConn3
  Three-Phase Parallel RLC Load59/LConn2 -- Three-Phase Transformer (Two Windings)59/RConn2
  Three-Phase Parallel RLC Load58/LConn2 -- Three-Phase Transformer (Two Windings)58/RConn2
  Three-Phase Parallel RLC Load59/LConn1 -- Three-Phase Transformer (Two Windings)59/RConn1
  Three-Phase Transformer (Two Windings)58/LConn2 -- B/RConn1 -- Three-Phase Transformer (Two Windings)59/LConn2
  Three-Phase Transformer (Two Windings)58/LConn1 -- A/RConn1 -- Three-Phase Transformer (Two Windings)59/LConn1
  Three-Phase Transformer (Two Windings)58/RConn1 -- Three-Phase Parallel RLC Load58/LConn3

== system FaultModel (1)/Subsystem16 ==
  Three-Phase Parallel RLC Load64 : powerlib/Elements/Three-Phase Parallel RLC Load  LConnTagsString=A|B|C  Configuration=Y (grounded)  NominalVoltage=33e3  Vabc=[1e3 1e3 1e3]  Vabcp=[1e3 1e3 1e3]  NominalFrequency=50  UnbalancedPower=off  ActivePower=40e6  InductivePower=100  CapacitivePower=100  Pabc=[10e3 9e3 11e3]  QLabc=[100 90 110]  QCabc=[100 90 110]  Pabcp=[10e3 9e3 11e3]  QLabcp=[100 90 110]  QCabcp=[100 90 110]  Measurements=None  LoadType=constant Z
  Three-Phase Parallel RLC Load65 : powerlib/Elements/Three-Phase Parallel RLC Load  LConnTagsString=A|B|C  Configuration=Y (grounded)  NominalVoltage=33e3  Vabc=[1e3 1e3 1e3]  Vabcp=[1e3 1e3 1e3]  NominalFrequency=50  UnbalancedPower=off  ActivePower=40e6  InductivePower=100  CapacitivePower=100  Pabc=[10e3 9e3 11e3]  QLabc=[100 90 110]  QCabc=[100 90 110]  Pabcp=[10e3 9e3 11e3]  QLabcp=[100 90 110]  QCabcp=[100 90 110]  Measurements=None  LoadType=constant Z
  Three-Phase Transformer (Two Windings)64 : powerlib/Elements/Three-Phase Transformer (Two Windings)  Winding1Connection=Delta (D1)  Winding2Connection=Yg  CoreType=Three single-phase transformers  SetSaturation=off  Hysteresis=off  DataFile='hysteresis'  SetInitialFlux=off  Measurements=None  UNITS=pu  NominalPower=[50e6 , 50 ]  Winding1=[ 132e3 , 0.002 , 0.08 ]  Winding2=[ 33e3 , 0.002 , 0.08 ]  Rm=500  Lm=500  L0=0.5  Saturation=[ 0,0 ; 0.0024,1.2 ; 1.0,1.52 ]  InitialFluxes=[ 0.8 , -0.8 , 0.7 ]  BreakLoop=off  DiscreteSolver=Trapezoidal iterative  DataType=off  TransfoNumber=1
  Three-Phase Transformer (Two Windings)65 : powerlib/Elements/Three-Phase Transformer (Two Windings)  Winding1Connection=Delta (D1)  Winding2Connection=Yg  CoreType=Three single-phase transformers  SetSaturation=off  Hysteresis=off  DataFile='hysteresis'  SetInitialFlux=off  Measurements=None  UNITS=pu  NominalPower=[50e6 , 50 ]  Winding1=[ 132e3 , 0.002 , 0.08 ]  Winding2=[ 33e3 , 0.002 , 0.08 ]  Rm=500  Lm=500  L0=0.5  Saturation=[ 0,0 ; 0.0024,1.2 ; 1.0,1.52 ]  InitialFluxes=[ 0.8 , -0.8 , 0.7 ]  BreakLoop=off  DiscreteSolver=Trapezoidal iterative  DataType=off  TransfoNumber=1
  A : PMIOPort  Side=Left
  B : PMIOPort  Port=2  Side=Left
  C : PMIOPort  Port=3  Side=Left
  connections:
  Three-Phase Transformer (Two Windings)64/LConn2 -- B/RConn1 -- Three-Phase Transformer (Two Windings)65/LConn2
  Three-Phase Parallel RLC Load65/LConn1 -- Three-Phase Transformer (Two Windings)65/RConn1
  Three-Phase Transformer (Two Windings)64/LConn3 -- C/RConn1 -- Three-Phase Transformer (Two Windings)65/LConn3
  Three-Phase Parallel RLC Load64/LConn1 -- Three-Phase Transformer (Two Windings)64/RConn3
  Three-Phase Parallel RLC Load65/LConn3 -- Three-Phase Transformer (Two Windings)65/RConn3
  Three-Phase Transformer (Two Windings)64/LConn1 -- A/RConn1 -- Three-Phase Transformer (Two Windings)65/LConn1
  Three-Phase Parallel RLC Load64/LConn2 -- Three-Phase Transformer (Two Windings)64/RConn2
  Three-Phase Parallel RLC Load65/LConn2 -- Three-Phase Transformer (Two Windings)65/RConn2
  Three-Phase Parallel RLC Load64/LConn3 -- Three-Phase Transformer (Two Windings)64/RConn1

== system FaultModel (1)/Subsystem17 ==
  Three-Phase Parallel RLC Load55 : powerlib/Elements/Three-Phase Parallel RLC Load  LConnTagsString=A|B|C  Configuration=Y (grounded)  NominalVoltage=33e3  Vabc=[1e3 1e3 1e3]  Vabcp=[1e3 1e3 1e3]  NominalFrequency=50  UnbalancedPower=off  ActivePower=60e6  InductivePower=100  CapacitivePower=100  Pabc=[10e3 9e3 11e3]  QLabc=[100 90 110]  QCabc=[100 90 110]  Pabcp=[10e3 9e3 11e3]  QLabcp=[100 90 110]  QCabcp=[100 90 110]  Measurements=None  LoadType=constant Z
  Three-Phase Parallel RLC Load56 : powerlib/Elements/Three-Phase Parallel RLC Load  LConnTagsString=A|B|C  Configuration=Y (grounded)  NominalVoltage=33e3  Vabc=[1e3 1e3 1e3]  Vabcp=[1e3 1e3 1e3]  NominalFrequency=50  UnbalancedPower=off  ActivePower=96e6  InductivePower=100  CapacitivePower=100  Pabc=[10e3 9e3 11e3]  QLabc=[100 90 110]  QCabc=[100 90 110]  Pabcp=[10e3 9e3 11e3]  QLabcp=[100 90 110]  QCabcp=[100 90 110]  Measurements=None  LoadType=constant Z
  Three-Phase Parallel RLC Load57 : powerlib/Elements/Three-Phase Parallel RLC Load  LConnTagsString=A|B|C  Configuration=Y (grounded)  NominalVoltage=33e3  Vabc=[1e3 1e3 1e3]  Vabcp=[1e3 1e3 1e3]  NominalFrequency=50  UnbalancedPower=off  ActivePower=40e6  InductivePower=100  CapacitivePower=100  Pabc=[10e3 9e3 11e3]  QLabc=[100 90 110]  QCabc=[100 90 110]  Pabcp=[10e3 9e3 11e3]  QLabcp=[100 90 110]  QCabcp=[100 90 110]  Measurements=None  LoadType=constant Z
  Three-Phase Transformer (Two Windings)55 : powerlib/Elements/Three-Phase Transformer (Two Windings)  Winding1Connection=Delta (D1)  Winding2Connection=Yg  CoreType=Three single-phase transformers  SetSaturation=off  Hysteresis=off  DataFile='hysteresis'  SetInitialFlux=off  Measurements=None  UNITS=pu  NominalPower=[75e6 , 50 ]  Winding1=[ 132e3 , 0.002 , 0.08 ]  Winding2=[ 33e3 , 0.002 , 0.08 ]  Rm=500  Lm=500  L0=0.5  Saturation=[ 0,0 ; 0.0024,1.2 ; 1.0,1.52 ]  InitialFluxes=[ 0.8 , -0.8 , 0.7 ]  BreakLoop=off  DiscreteSolver=Trapezoidal iterative  DataType=off  TransfoNumber=1
  Three-Phase Transformer (Two Windings)56 : powerlib/Elements/Three-Phase Transformer (Two Windings)  Winding1Connection=Delta (D1)  Winding2Connection=Yg  CoreType=Three single-phase transformers  SetSaturation=off  Hysteresis=off  DataFile='hysteresis'  SetInitialFlux=off  Measurements=None  UNITS=pu  NominalPower=[120e6 , 50 ]  Winding1=[ 132e3 , 0.002 , 0.08 ]  Winding2=[ 33e3 , 0.002 , 0.08 ]  Rm=500  Lm=500  L0=0.5  Saturation=[ 0,0 ; 0.0024,1.2 ; 1.0,1.52 ]  InitialFluxes=[ 0.8 , -0.8 , 0.7 ]  BreakLoop=off  DiscreteSolver=Trapezoidal iterative  DataType=off  TransfoNumber=1
  Three-Phase Transformer (Two Windings)57 : powerlib/Elements/Three-Phase Transformer (Two Windings)  Winding1Connection=Delta (D1)  Winding2Connection=Yg  CoreType=Three single-phase transformers  SetSaturation=off  Hysteresis=off  DataFile='hysteresis'  SetInitialFlux=off  Measurements=None  UNITS=pu  NominalPower=[50e6 , 50 ]  Winding1=[ 132e3 , 0.002 , 0.08 ]  Winding2=[ 33e3 , 0.002 , 0.08 ]  Rm=500  Lm=500  L0=0.5  Saturation=[ 0,0 ; 0.0024,1.2 ; 1.0,1.52 ]  InitialFluxes=[ 0.8 , -0.8 , 0.7 ]  BreakLoop=off  DiscreteSolver=Trapezoidal iterative  DataType=off  TransfoNumber=1
  A : PMIOPort  Side=Left
  B : PMIOPort  Port=2  Side=Left
  C : PMIOPort  Port=3  Side=Left
  connections:
  Three-Phase Parallel RLC Load57/LConn3 -- Three-Phase Transformer (Two Windings)57/RConn3
  Three-Phase Parallel RLC Load55/LConn2 -- Three-Phase Transformer (Two Windings)55/RConn2
  Three-Phase Parallel RLC Load55/LConn1 -- Three-Phase Transformer (Two Windings)55/RConn1
  Three-Phase Parallel RLC Load57/LConn1 -- Three-Phase Transformer (Two Windings)57/RConn1
  Three-Phase Parallel RLC Load56/LConn2 -- Three-Phase Transformer (Two Windings)56/RConn2
  Three-Phase Parallel RLC Load56/LConn1 -- Three-Phase Transformer (Two Windings)56/RConn1
  Three-Phase Parallel RLC Load57/LConn2 -- Three-Phase Transformer (Two Windings)57/RConn2
  Three-Phase Parallel RLC Load56/LConn3 -- Three-Phase Transformer (Two Windings)56/RConn3
  Three-Phase Parallel RLC Load55/LConn3 -- Three-Phase Transformer (Two Windings)55/RConn3
  Three-Phase Transformer (Two Windings)57/LConn1 -- A/RConn1 -- Three-Phase Transformer (Two Windings)55/LConn1 -- Three-Phase Transformer (Two Windings)56/LConn1
  Three-Phase Transformer (Two Windings)57/LConn2 -- Three-Phase Transformer (Two Windings)56/LConn2 -- B/RConn1 -- Three-Phase Transformer (Two Windings)55/LConn2
  Three-Phase Transformer (Two Windings)57/LConn3 -- Three-Phase Transformer (Two Windings)55/LConn3 -- C/RConn1 -- Three-Phase Transformer (Two Windings)56/LConn3

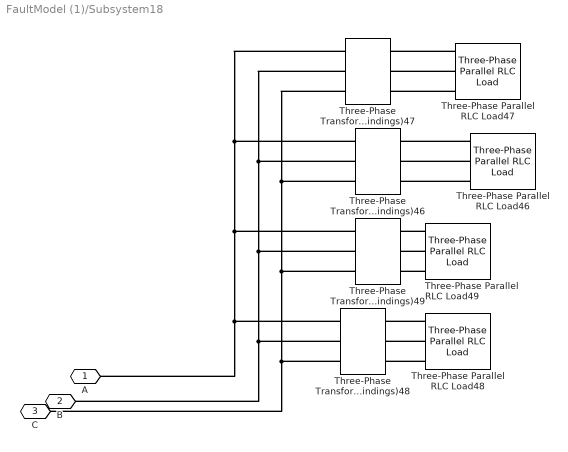
== system FaultModel (1)/Subsystem18 ==
  Three-Phase Parallel RLC Load46 : powerlib/Elements/Three-Phase Parallel RLC Load  LConnTagsString=A|B|C  Configuration=Y (grounded)  NominalVoltage=33e3  Vabc=[1e3 1e3 1e3]  Vabcp=[1e3 1e3 1e3]  NominalFrequency=50  UnbalancedPower=off  ActivePower=60e6  InductivePower=100  CapacitivePower=100  Pabc=[10e3 9e3 11e3]  QLabc=[100 90 110]  QCabc=[100 90 110]  Pabcp=[10e3 9e3 11e3]  QLabcp=[100 90 110]  QCabcp=[100 90 110]  Measurements=None  LoadType=constant Z
  Three-Phase Parallel RLC Load47 : powerlib/Elements/Three-Phase Parallel RLC Load  LConnTagsString=A|B|C  Configuration=Y (grounded)  NominalVoltage=33e3  Vabc=[1e3 1e3 1e3]  Vabcp=[1e3 1e3 1e3]  NominalFrequency=50  UnbalancedPower=off  ActivePower=60e6  InductivePower=100  CapacitivePower=100  Pabc=[10e3 9e3 11e3]  QLabc=[100 90 110]  QCabc=[100 90 110]  Pabcp=[10e3 9e3 11e3]  QLabcp=[100 90 110]  QCabcp=[100 90 110]  Measurements=None  LoadType=constant Z
  Three-Phase Parallel RLC Load48 : powerlib/Elements/Three-Phase Parallel RLC Load  LConnTagsString=A|B|C  Configuration=Y (grounded)  NominalVoltage=33e3  Vabc=[1e3 1e3 1e3]  Vabcp=[1e3 1e3 1e3]  NominalFrequency=50  UnbalancedPower=off  ActivePower=96e6  InductivePower=100  CapacitivePower=100  Pabc=[10e3 9e3 11e3]  QLabc=[100 90 110]  QCabc=[100 90 110]  Pabcp=[10e3 9e3 11e3]  QLabcp=[100 90 110]  QCabcp=[100 90 110]  Measurements=None  LoadType=constant Z
  Three-Phase Parallel RLC Load49 : powerlib/Elements/Three-Phase Parallel RLC Load  LConnTagsString=A|B|C  Configuration=Y (grounded)  NominalVoltage=33e3  Vabc=[1e3 1e3 1e3]  Vabcp=[1e3 1e3 1e3]  NominalFrequency=50  UnbalancedPower=off  ActivePower=96e6  InductivePower=100  CapacitivePower=100  Pabc=[10e3 9e3 11e3]  QLabc=[100 90 110]  QCabc=[100 90 110]  Pabcp=[10e3 9e3 11e3]  QLabcp=[100 90 110]  QCabcp=[100 90 110]  Measurements=None  LoadType=constant Z
  Three-Phase Transformer (Two Windings)46 : powerlib/Elements/Three-Phase Transformer (Two Windings)  Winding1Connection=Delta (D1)  Winding2Connection=Yg  CoreType=Three single-phase transformers  SetSaturation=off  Hysteresis=off  DataFile='hysteresis'  SetInitialFlux=off  Measurements=None  UNITS=pu  NominalPower=[75e6 , 50 ]  Winding1=[ 132e3 , 0.002 , 0.08 ]  Winding2=[ 33e3 , 0.002 , 0.08 ]  Rm=500  Lm=500  L0=0.5  Saturation=[ 0,0 ; 0.0024,1.2 ; 1.0,1.52 ]  InitialFluxes=[ 0.8 , -0.8 , 0.7 ]  BreakLoop=off  DiscreteSolver=Trapezoidal iterative  DataType=off  TransfoNumber=1
  Three-Phase Transformer (Two Windings)47 : powerlib/Elements/Three-Phase Transformer (Two Windings)  Winding1Connection=Delta (D1)  Winding2Connection=Yg  CoreType=Three single-phase transformers  SetSaturation=off  Hysteresis=off  DataFile='hysteresis'  SetInitialFlux=off  Measurements=None  UNITS=pu  NominalPower=[75e6 , 50 ]  Winding1=[ 132e3 , 0.002 , 0.08 ]  Winding2=[ 33e3 , 0.002 , 0.08 ]  Rm=500  Lm=500  L0=0.5  Saturation=[ 0,0 ; 0.0024,1.2 ; 1.0,1.52 ]  InitialFluxes=[ 0.8 , -0.8 , 0.7 ]  BreakLoop=off  DiscreteSolver=Trapezoidal iterative  DataType=off  TransfoNumber=1
  Three-Phase Transformer (Two Windings)48 : powerlib/Elements/Three-Phase Transformer (Two Windings)  Winding1Connection=Delta (D1)  Winding2Connection=Yg  CoreType=Three single-phase transformers  SetSaturation=off  Hysteresis=off  DataFile='hysteresis'  SetInitialFlux=off  Measurements=None  UNITS=pu  NominalPower=[120e6 , 50 ]  Winding1=[ 132e3 , 0.002 , 0.08 ]  Winding2=[ 33e3 , 0.002 , 0.08 ]  Rm=500  Lm=500  L0=0.5  Saturation=[ 0,0 ; 0.0024,1.2 ; 1.0,1.52 ]  InitialFluxes=[ 0.8 , -0.8 , 0.7 ]  BreakLoop=off  DiscreteSolver=Trapezoidal iterative  DataType=off  TransfoNumber=1
  Three-Phase Transformer (Two Windings)49 : powerlib/Elements/Three-Phase Transformer (Two Windings)  Winding1Connection=Delta (D1)  Winding2Connection=Yg  CoreType=Three single-phase transformers  SetSaturation=off  Hysteresis=off  DataFile='hysteresis'  SetInitialFlux=off  Measurements=None  UNITS=pu  NominalPower=[120e6 , 50 ]  Winding1=[ 132e3 , 0.002 , 0.08 ]  Winding2=[ 33e3 , 0.002 , 0.08 ]  Rm=500  Lm=500  L0=0.5  Saturation=[ 0,0 ; 0.0024,1.2 ; 1.0,1.52 ]  InitialFluxes=[ 0.8 , -0.8 , 0.7 ]  BreakLoop=off  DiscreteSolver=Trapezoidal iterative  DataType=off  TransfoNumber=1
  A : PMIOPort  Side=Left
  B : PMIOPort  Port=2  Side=Left
  C : PMIOPort  Port=3  Side=Left
  connections:
  Three-Phase Parallel RLC Load46/LConn3 -- Three-Phase Transformer (Two Windings)46/RConn3
  Three-Phase Transformer (Two Windings)47/LConn3 -- C/RConn1 -- Three-Phase Transformer (Two Windings)48/LConn3 -- Three-Phase Transformer (Two Windings)49/LConn3 -- Three-Phase Transformer (Two Windings)46/LConn3
  Three-Phase Parallel RLC Load47/LConn1 -- Three-Phase Transformer (Two Windings)47/RConn1
  Three-Phase Transformer (Two Windings)49/LConn1 -- Three-Phase Transformer (Two Windings)47/LConn1 -- Three-Phase Transformer (Two Windings)46/LConn1 -- A/RConn1 -- Three-Phase Transformer (Two Windings)48/LConn1
  Three-Phase Parallel RLC Load48/LConn1 -- Three-Phase Transformer (Two Windings)48/RConn1
  Three-Phase Parallel RLC Load49/LConn1 -- Three-Phase Transformer (Two Windings)49/RConn1
  Three-Phase Transformer (Two Windings)49/LConn2 -- Three-Phase Transformer (Two Windings)47/LConn2 -- Three-Phase Transformer (Two Windings)46/LConn2 -- B/RConn1 -- Three-Phase Transformer (Two Windings)48/LConn2
  Three-Phase Parallel RLC Load47/LConn2 -- Three-Phase Transformer (Two Windings)47/RConn2
  Three-Phase Parallel RLC Load46/LConn2 -- Three-Phase Transformer (Two Windings)46/RConn2
  Three-Phase Parallel RLC Load48/LConn3 -- Three-Phase Transformer (Two Windings)48/RConn3
  Three-Phase Parallel RLC Load47/LConn3 -- Three-Phase Transformer (Two Windings)47/RConn3
  Three-Phase Parallel RLC Load48/LConn2 -- Three-Phase Transformer (Two Windings)48/RConn2
  Three-Phase Parallel RLC Load46/LConn1 -- Three-Phase Transformer (Two Windings)46/RConn1
  Three-Phase Parallel RLC Load49/LConn3 -- Three-Phase Transformer (Two Windings)49/RConn3
  Three-Phase Parallel RLC Load49/LConn2 -- Three-Phase Transformer (Two Windings)49/RConn2

== system FaultModel (1)/Subsystem19 ==
  Three-Phase Parallel RLC Load68 : powerlib/Elements/Three-Phase Parallel RLC Load  LConnTagsString=A|B|C  Configuration=Y (grounded)  NominalVoltage=33e3  Vabc=[1e3 1e3 1e3]  Vabcp=[1e3 1e3 1e3]  NominalFrequency=50  UnbalancedPower=off  ActivePower=60e6  InductivePower=100  CapacitivePower=100  Pabc=[10e3 9e3 11e3]  QLabc=[100 90 110]  QCabc=[100 90 110]  Pabcp=[10e3 9e3 11e3]  QLabcp=[100 90 110]  QCabcp=[100 90 110]  Measurements=None  LoadType=constant Z
  Three-Phase Parallel RLC Load69 : powerlib/Elements/Three-Phase Parallel RLC Load  LConnTagsString=A|B|C  Configuration=Y (grounded)  NominalVoltage=33e3  Vabc=[1e3 1e3 1e3]  Vabcp=[1e3 1e3 1e3]  NominalFrequency=50  UnbalancedPower=off  ActivePower=60e6  InductivePower=100  CapacitivePower=100  Pabc=[10e3 9e3 11e3]  QLabc=[100 90 110]  QCabc=[100 90 110]  Pabcp=[10e3 9e3 11e3]  QLabcp=[100 90 110]  QCabcp=[100 90 110]  Measurements=None  LoadType=constant Z
  Three-Phase Transformer (Two Windings)68 : powerlib/Elements/Three-Phase Transformer (Two Windings)  Winding1Connection=Delta (D1)  Winding2Connection=Yg  CoreType=Three single-phase transformers  SetSaturation=off  Hysteresis=off  DataFile='hysteresis'  SetInitialFlux=off  Measurements=None  UNITS=pu  NominalPower=[75e6 , 50 ]  Winding1=[ 132e3 , 0.002 , 0.08 ]  Winding2=[ 33e3 , 0.002 , 0.08 ]  Rm=500  Lm=500  L0=0.5  Saturation=[ 0,0 ; 0.0024,1.2 ; 1.0,1.52 ]  InitialFluxes=[ 0.8 , -0.8 , 0.7 ]  BreakLoop=off  DiscreteSolver=Trapezoidal iterative  DataType=off  TransfoNumber=1
  Three-Phase Transformer (Two Windings)69 : powerlib/Elements/Three-Phase Transformer (Two Windings)  Winding1Connection=Delta (D1)  Winding2Connection=Yg  CoreType=Three single-phase transformers  SetSaturation=off  Hysteresis=off  DataFile='hysteresis'  SetInitialFlux=off  Measurements=None  UNITS=pu  NominalPower=[75e6 , 50 ]  Winding1=[ 132e3 , 0.002 , 0.08 ]  Winding2=[ 33e3 , 0.002 , 0.08 ]  Rm=500  Lm=500  L0=0.5  Saturation=[ 0,0 ; 0.0024,1.2 ; 1.0,1.52 ]  InitialFluxes=[ 0.8 , -0.8 , 0.7 ]  BreakLoop=off  DiscreteSolver=Trapezoidal iterative  DataType=off  TransfoNumber=1
  A : PMIOPort  Side=Left
  B : PMIOPort  Port=2  Side=Left
  C : PMIOPort  Port=3  Side=Left
  connections:
  Three-Phase Transformer (Two Windings)68/LConn3 -- C/RConn1 -- Three-Phase Transformer (Two Windings)69/LConn3
  Three-Phase Transformer (Two Windings)68/LConn1 -- A/RConn1 -- Three-Phase Transformer (Two Windings)69/LConn1
  Three-Phase Transformer (Two Windings)69/LConn2 -- B/RConn1 -- Three-Phase Transformer (Two Windings)68/LConn2
  Three-Phase Parallel RLC Load68/LConn3 -- Three-Phase Transformer (Two Windings)68/RConn3
  Three-Phase Parallel RLC Load69/LConn1 -- Three-Phase Transformer (Two Windings)69/RConn1
  Three-Phase Parallel RLC Load69/LConn2 -- Three-Phase Transformer (Two Windings)69/RConn2
  Three-Phase Parallel RLC Load68/LConn1 -- Three-Phase Transformer (Two Windings)68/RConn1
  Three-Phase Parallel RLC Load69/LConn3 -- Three-Phase Transformer (Two Windings)69/RConn3
  Three-Phase Parallel RLC Load68/LConn2 -- Three-Phase Transformer (Two Windings)68/RConn2
